simulink model "Control_propulsion_realista"  (R2024b)
settings: Solver=FixedStepAuto  StartTime=0.0  StopTime=tf  FixedStep=50  MaxStep=25  MinStep=1  RelTol=1e-10  AbsTol=1e-10
values from neighbouring files (symbols this model uses):
  v_2 = [-14.5213651902 22.4460020945 10.2931913359]    [datos_trayectoria_mejorada.mat]
undefined symbols (not defined in the file or in its folder): duracion_propul, endDate, F_control, F_quimico, Isp_control, Isp_quimico, m_final, m_i, m_propulsor_quimico, startDate1, ultimo_Tiempo
libraries: simulink x5
settings Model: SimulationMode=rapid-accelerator  Creator=user  LastModifiedBy=benit
settings SolverCC: AutoScaleAbsTol=off  InitialStep=25

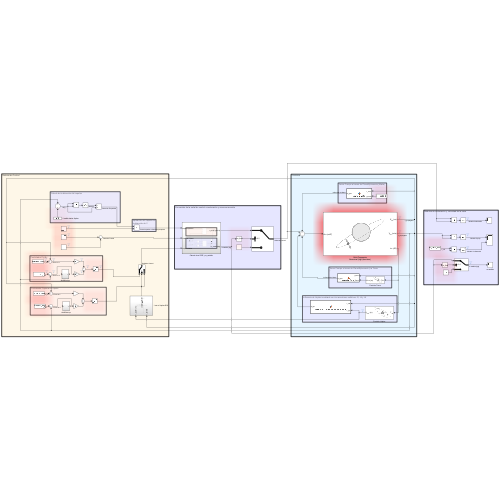
[thumbnail: Simulink's stored preview of the top-level diagram]
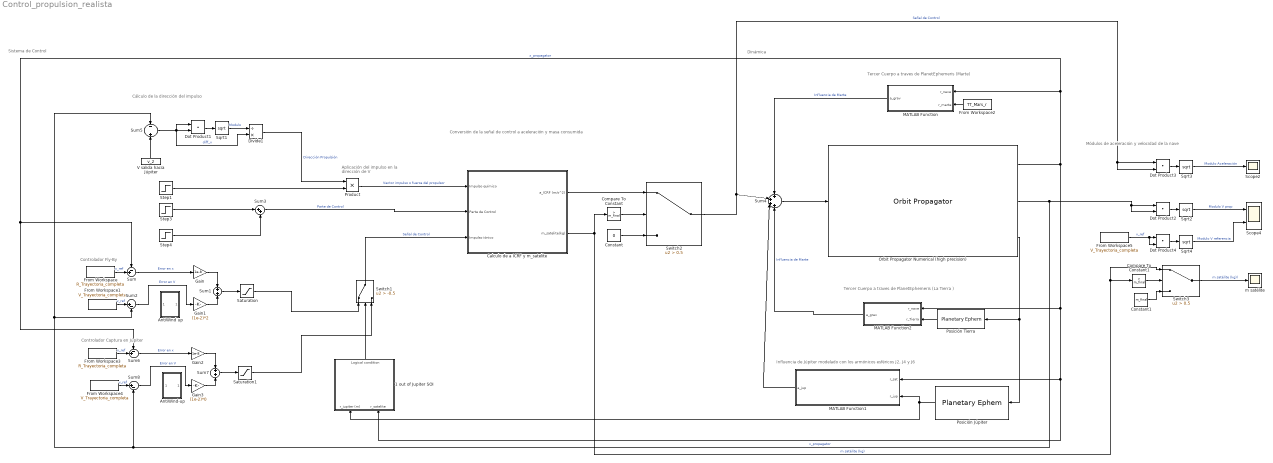
== system Control_propulsion_realista ==
  note: Dinámica
  note: Conversión de la señal de control a aceleración y masa consumida
  note: Sistema de Control
  note: Módulos de aceleración y velocidad de la nave
  note: Controlador Fly-By
  note: Controlador Captura en Júpiter
  note: Influencia de Júpiter modelado con los armónicos esféricos J2, J4 y J6
  note: Cálculo de la dirección del impulso
  note: Tercer Cuerpo a traves de PlanetEphemeris (Marte)
  note: Aplicación del impulso en
      | la dirección de V
  note: Tercer Cuerpo a traves de PlanetEphemeris (La Tierra
      | )
  1 out of Jupiter SOI : Subsystem
  AntiWind up : Subsystem
  AntiWind-up : Subsystem
  Calculo de a ICRF y m_satelite : Subsystem
  Compare To Constant : simulink/Logic and Bit Operations/Compare To Constant  relop=>  const=m_final  OutDataTypeStr=boolean
  Compare To Constant1 : simulink/Logic and Bit Operations/Compare To Constant  relop=>  const=m_final  OutDataTypeStr=boolean
  Constant : Constant  Value=0
  Constant1 : Constant  Value=m_final
  Divide1 : Product  Inputs=/*
  Dot Product{1..4} (4 alike) : DotProduct  OutDataTypeStr=Inherit: Inherit via internal rule
  From Workspace : FromWorkspace  VariableName=R_Trayectoria_completa
  From Workspace1 : FromWorkspace  VariableName=V_Trayectoria_completa
  From Workspace2 : FromWorkspace  VariableName=TT_Mars_r
  From Workspace3 : FromWorkspace  VariableName=R_Trayectoria_completa
  From Workspace4 : FromWorkspace  VariableName=V_Trayectoria_completa
  From Workspace5 : FromWorkspace  VariableName=V_Trayectoria_completa
  Gain : Gain  Gain=1e-8
  Gain1 : Gain  Gain=(1e-2)*2
  Gain2 : Gain  Gain=1e-8
  Gain3 : Gain  Gain=(1e-2)*0
  MATLAB Function : MATLAB Function  TreatAsAtomicUnit=on
  MATLAB Function1 : MATLAB Function  TreatAsAtomicUnit=on
  MATLAB Function2 : MATLAB Function  TreatAsAtomicUnit=on
  Orbit Propagator Numerical (high precision) : OrbitPropagator  propagator=Numerical (high precision)  accelIn=on  startDate=startDate1  semiMajorAxis=sma  eccentricity=ecc  inclination=inc  raan=RAAN  argPeriapsis=aop  trueAnomaly=true_an  inertialPosition=[3649700.0 3308200.0 -4676600.0]  inertialVelocity=[-2750.8 6666.4 2573.4]  fixedPosition=[-4142689.0 -2676864.7 -4669861.6]  fixedVelocity=[1452.7 -6720.7 2568.1]  centralBody=Sun  customR=3396200  customMu=4.305e13  customJ2=1.0826269e-03  customOmega=4.06125949e-3  useEphemerisDateRange=off  ephemerisStartDate=startDate2  ephemerisEndDate=startDate1+tf  includeEarthGravity=off  includeMoonGravity=off  includeJupiterGravity=on
  Posición Júpiter : PlanetaryEphem  units=m,m/s  center=Sun  target=Jupiter  startDate=startDate2  endDate=endDate*1.02  outputVelocity=off
  Posición Tierra : PlanetaryEphem  units=m,m/s  center=Sun  target=Earth  startDate=startDate2  endDate=endDate*1.02  outputVelocity=off
  Product : Product
  Saturation : Saturate  UpperLimit=F_control  LowerLimit=-F_control
  Saturation1 : Saturate  UpperLimit=F_control  LowerLimit=-F_control
  Scope2 : Scope
  Scope4 : Scope  NumInputPorts=2
  Sqrt{1..4} (4 alike) : Sqrt
  Step1 : Step  Time=ultimo_Tiempo+duracion_propul  Before=F_quimico  After=0  SampleTime=0
  Step3 : Step  Time=ultimo_Tiempo  SampleTime=0
  Step4 : Step  Time=ultimo_Tiempo+duracion_propul  After=-1  SampleTime=0
  Sum : Sum  Inputs=-+|
  Sum1 : Sum  Inputs=+|+
  Sum2 : Sum  Inputs=|+-
  Sum3 : Sum  Inputs=|++
  Sum4 : Sum  Inputs=++++
  Sum5 : Sum  Inputs=-+
  Sum6 : Sum  Inputs=-+|
  Sum7 : Sum  Inputs=+|+
  Sum8 : Sum  Inputs=|+-
  Switch1 : Switch  Criteria=u2 > Threshold  Threshold=-0.5  SaturateOnIntegerOverflow=off  InputSameDT=off
  Switch2 : Switch  Criteria=u2 > Threshold  Threshold=0.5  SaturateOnIntegerOverflow=off  InputSameDT=off
  Switch3 : Switch  Criteria=u2 > Threshold  Threshold=0.5  SaturateOnIntegerOverflow=off  InputSameDT=off
  V salida hacia Júpiter : Constant  Value=v_2
  m satélite : Scope
  wires:
  Sum/1 -> Gain/1  "Error en x"
  From Workspace/1 -> Sum/2  "x_ref"
  Orbit Propagator Numerical (high precision)/1 -> Sum6/1, Sum/1, MATLAB Function/1(r_nave), MATLAB Function1/1(r_sat), 1 out of Jupiter SOI/2(r_satelite), MATLAB Function2/1(r_nave)  "x_propagator"
  Gain/1 -> Sum1/1
  From Workspace1/1 -> Sum2/1  "v_ref"
  Gain1/1 -> Sum1/2
  Sum1/1 -> Saturation/1
  Step1/1 -> Product/2
  Step3/1 -> Sum3/1
  Sum4/1 -> Orbit Propagator Numerical (high precision)/1
  Step4/1 -> Sum3/2
  Product/1 -> Calculo de a ICRF y m_satelite/1(Impulso químico)  "Vector impulso o fuerza del propulsor"
  From Workspace2/1 -> MATLAB Function/2(r_marte)
  V salida hacia Júpiter/1 -> Sum5/2
  Sum5/1 -> Dot Product1/1, Divide1/2, Dot Product1/2  "diff_v"
  Sqrt1/1 -> Divide1/1  "Modulo"
  Dot Product1/1 -> Sqrt1/1
  Divide1/1 -> Product/1  "Dirección Propulsión"
  Sum3/1 -> Calculo de a ICRF y m_satelite/2(Parte de Control)  "Parte de Control"
  MATLAB Function/1(a_grav) -> Sum4/1  "Influencia de Marte"
  Orbit Propagator Numerical (high precision)/3 -> Posición Tierra/1, Posición Júpiter/1
  Posición Júpiter/1 -> MATLAB Function1/2(r_jup), 1 out of Jupiter SOI/1(r_jupiter (m))
  From Workspace3/1 -> Sum6/2  "x_ref"
  Sum7/1 -> Saturation1/1
  From Workspace4/1 -> Sum8/1  "v_ref"
  Gain2/1 -> Sum7/1
  Gain3/1 -> Sum7/2
  Sum6/1 -> Gain2/1  "Error en x"
  Orbit Propagator Numerical (high precision)/2 -> Dot Product2/2, Dot Product2/1, Sum2/2, Sum5/1, Sum8/2  "v_propagator"
  Saturation/1 -> Switch1/1
  Saturation1/1 -> Switch1/3
  Switch1/1 -> Calculo de a ICRF y m_satelite/3(Impulso iónico)  "Señal de Control"
  Calculo de a ICRF y m_satelite/2(m_satelite(kg)) -> Switch3/1, Compare To Constant1/1, Compare To Constant/1  "m satélite (kg)"
  Dot Product2/1 -> Sqrt2/1
  Sqrt2/1 -> Scope4/1  "Modulo V prop"
  Sqrt3/1 -> Scope2/1  "Modulo Aceleración"
  Dot Product3/1 -> Sqrt3/1
  Sqrt4/1 -> Scope4/2  "Modulo V referencia"
  Dot Product4/1 -> Sqrt4/1
  From Workspace5/1 -> Dot Product4/2, Dot Product4/1  "v_ref"
  MATLAB Function1/1(a_jup) -> Sum4/3
  Switch2/1 -> Dot Product3/2, Dot Product3/1, Sum4/2  "Señal de Control"
  Calculo de a ICRF y m_satelite/1(a_ICRF (m/s^2)) -> Switch2/1
  Constant/1 -> Switch2/3
  Compare To Constant/1 -> Switch2/2
  Compare To Constant1/1 -> Switch3/2
  Constant1/1 -> Switch3/3
  Switch3/1 -> m satélite/1  "m satélite (kg)l"
  1 out of Jupiter SOI/1("Logical condition ") -> Switch1/2
  Posición Tierra/1 -> MATLAB Function2/2(r_Tierra)
  Sum2/1 -> Gain1/1  "Error en V"
  Sum8/1 -> Gain3/1  "Error en V"
  MATLAB Function2/1(a_grav) -> Sum4/4  "Influencia de Marte"

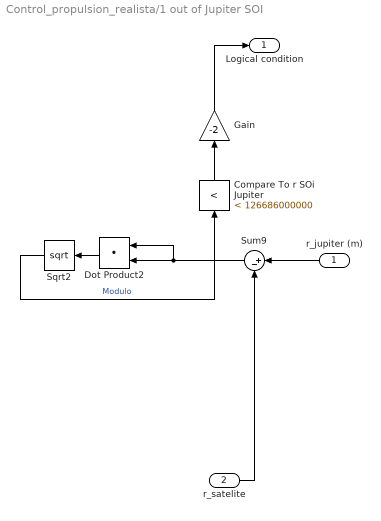
== system Control_propulsion_realista/1 out of Jupiter SOI ==
  r_jupiter (m) : Inport
  r_satelite : Inport  Port=2
  Compare To r SOi Jupiter : simulink/Logic and Bit Operations/Compare To Constant  relop=<  const=126686000000  OutDataTypeStr=boolean
  Dot Product2 : DotProduct  OutDataTypeStr=Inherit: Inherit via internal rule
  Gain : Gain  Gain=-2
  Sqrt2 : Sqrt
  Sum9 : Sum  Inputs=|+-
  "Logical condition " : Outport
  wires:
  Dot Product2/1 -> Sqrt2/1
  r_satelite/1 -> Sum9/2
  Compare To r SOi Jupiter/1 -> Gain/1
  Sqrt2/1 -> Compare To r SOi Jupiter/1  "Modulo"
  r_jupiter (m)/1 -> Sum9/1
  Sum9/1 -> Dot Product2/2, Dot Product2/1
  Gain/1 -> "Logical condition "/1

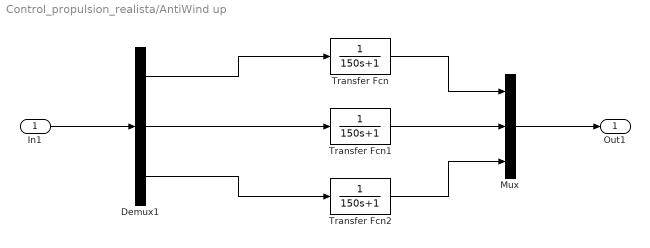
== system Control_propulsion_realista/AntiWind up ==
  In1 : Inport
  Demux1 : Demux  Outputs=3
  Mux : Mux  Inputs=3
  Transfer Fcn : TransferFcn  Denominator=[150 1]
  Transfer Fcn1 : TransferFcn  Denominator=[150 1]
  Transfer Fcn2 : TransferFcn  Denominator=[150 1]
  Out1 : Outport
  wires:
  Demux1/1 -> Transfer Fcn/1
  Demux1/2 -> Transfer Fcn1/1
  Demux1/3 -> Transfer Fcn2/1
  Transfer Fcn/1 -> Mux/1
  Transfer Fcn1/1 -> Mux/2
  Transfer Fcn2/1 -> Mux/3
  Mux/1 -> Out1/1
  In1/1 -> Demux1/1

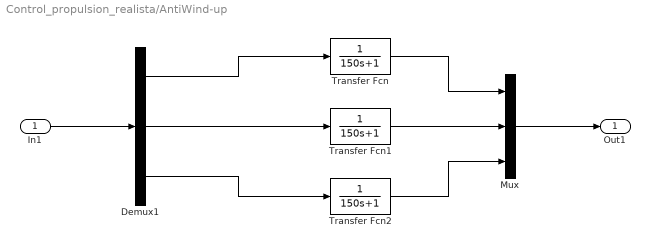
== system Control_propulsion_realista/AntiWind-up ==
  In1 : Inport
  Demux1 : Demux  Outputs=3
  Mux : Mux  Inputs=3
  Transfer Fcn : TransferFcn  Denominator=[150 1]
  Transfer Fcn1 : TransferFcn  Denominator=[150 1]
  Transfer Fcn2 : TransferFcn  Denominator=[150 1]
  Out1 : Outport
  wires:
  Demux1/1 -> Transfer Fcn/1
  Demux1/2 -> Transfer Fcn1/1
  Demux1/3 -> Transfer Fcn2/1
  Transfer Fcn/1 -> Mux/1
  Transfer Fcn1/1 -> Mux/2
  Transfer Fcn2/1 -> Mux/3
  Mux/1 -> Out1/1
  In1/1 -> Demux1/1

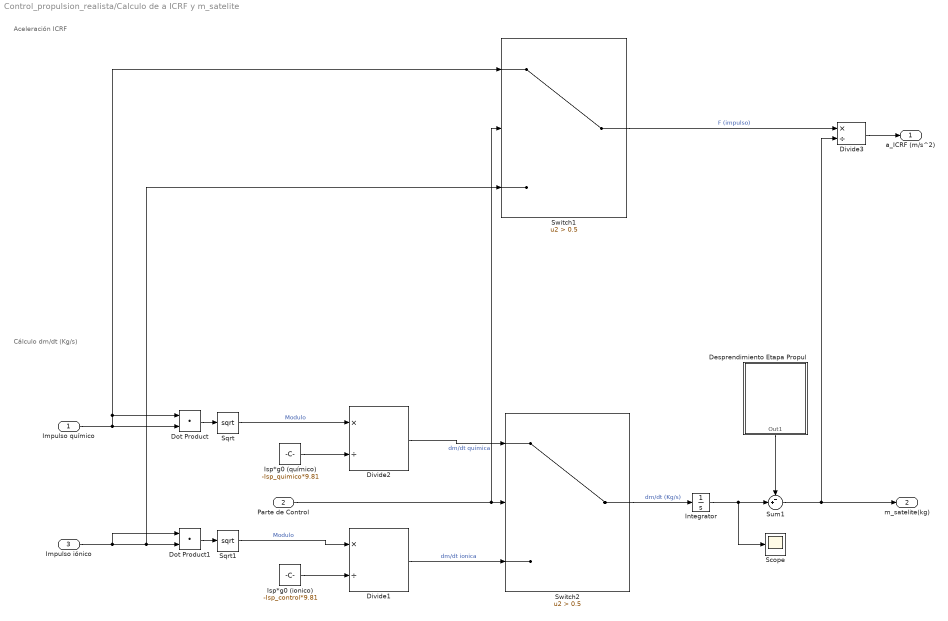
== system Control_propulsion_realista/Calculo de a ICRF y m_satelite ==
  note: Aceleración ICRF
  note: Cálculo dm/dt (Kg/s)
  Impulso químico : Inport
  Parte de Control : Inport  Port=2
  Impulso iónico : Inport  Port=3
  Desprendimiento Etapa Propul : Subsystem
  Divide1 : Product  Inputs=*/
  Divide2 : Product  Inputs=*/
  Divide3 : Product  Inputs=*/
  Dot Product : DotProduct  OutDataTypeStr=Inherit: Inherit via internal rule
  Dot Product1 : DotProduct  OutDataTypeStr=Inherit: Inherit via internal rule
  Integrator : Integrator  InitialCondition=m_i
  Isp*g0 (ionico) : Constant  Value=-Isp_control*9.81
  Isp*g0 (químico) : Constant  Value=-Isp_quimico*9.81
  Scope : Scope
  Sqrt : Sqrt
  Sqrt1 : Sqrt
  Sum1 : Sum  Inputs=-+|
  Switch1 : Switch  Criteria=u2 > Threshold  Threshold=0.5  SaturateOnIntegerOverflow=off  InputSameDT=off
  Switch2 : Switch  Criteria=u2 > Threshold  Threshold=0.5  SaturateOnIntegerOverflow=off  InputSameDT=off
  a_ICRF (m/s^2) : Outport
  m_satelite(kg) : Outport  Port=2
  wires:
  Parte de Control/1 -> Switch1/2, Switch2/2
  Divide2/1 -> Switch2/1  "dm/dt química"
  Isp*g0 (químico)/1 -> Divide2/2
  Isp*g0 (ionico)/1 -> Divide1/2
  Divide1/1 -> Switch2/3  "dm/dt ionica"
  Switch2/1 -> Integrator/1  "dm/dt (Kg/s)"
  Dot Product/1 -> Sqrt/1
  Impulso químico/1 -> Switch1/1, Dot Product/1, Dot Product/2
  Sqrt/1 -> Divide2/1  "Modulo"
  Dot Product1/1 -> Sqrt1/1
  Sqrt1/1 -> Divide1/1  "Modulo"
  Impulso iónico/1 -> Switch1/3, Dot Product1/2, Dot Product1/1
  Switch1/1 -> Divide3/1  "F (impulso)"
  Divide3/1 -> a_ICRF (m/s^2)/1
  Integrator/1 -> Scope/1, Sum1/2
  Desprendimiento Etapa Propul/1(Out1) -> Sum1/1
  Sum1/1 -> Divide3/2, m_satelite(kg)/1

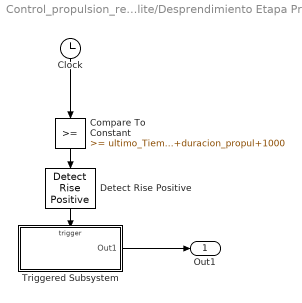
== system Control_propulsion_realista/Calculo de a ICRF y m_satelite/Desprendimiento Etapa Propul ==
  Clock : Clock
  Compare To Constant : simulink/Logic and Bit Operations/Compare To Constant  relop=>=  const=ultimo_Tiempo+duracion_propul+1000  OutDataTypeStr=boolean
  Detect Rise Positive : simulink/Logic and Bit Operations/Detect Rise Positive  vinit=0  OutDataTypeStr=boolean
  Triggered Subsystem : Subsystem  TreatAsAtomicUnit=on
  Out1 : Outport
  wires:
  Clock/1 -> Compare To Constant/1
  Detect Rise Positive/1 -> Triggered Subsystem/Trigger
  Compare To Constant/1 -> Detect Rise Positive/1
  Triggered Subsystem/1(Out1) -> Out1/1

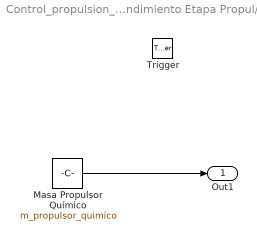
== system Control_propulsion_realista/Calculo de a ICRF y m_satelite/Desprendimiento Etapa Propul/Triggered Subsystem ==
  Trigger : TriggerPort  VariantControl=(inherit)
  Masa Propulsor Químico : Constant  Value=m_propulsor_quimico
  Out1 : Outport
  wires:
  Masa Propulsor Químico/1 -> Out1/1

== matlab function Control_propulsion_realista/MATLAB Function ==
  data: r_nave input; a_grav output; r_marte input
function a_grav = gravedadMarte(r_nave, r_marte)
%#codegen

% Constante gravitacional de Marte
mu_marte = 4.282837e13; % [m^3/s^2]

% Vector relativo
r_rel = r_nave - r_marte;

% Magnitud de la distancia
dist = norm(r_rel);

% Aceleración gravitatoria
a_grav = (-mu_marte / dist^3) * r_rel;

end

== matlab function Control_propulsion_realista/MATLAB Function2 ==
  data: r_nave input; a_grav output; r_Tierra input
function a_grav = gravedadTierra(r_nave, r_Tierra)
%#codegen

% Constante gravitacional de Marte
mu_marte = 3.986e14; % [m^3/s^2]

% Vector relativo
r_rel = r_nave - r_Tierra;

% Magnitud de la distancia
dist = norm(r_rel);

% Aceleración gravitatoria
a_grav = (-mu_marte / dist^3) * r_rel;

end

== matlab function Control_propulsion_realista/MATLAB Function1 ==
  data: r_sat input; a_jup output; r_jup input
function a_jup = aceleracion_jupiter_armonicos_simulink(r_sat, r_jup)
    % Entradas y salidas en metros / segundos
    % r_sat, r_jup: [3x1] vectores de posición en metros

    % Constantes de Júpiter (SI)
    mu_jup = 1.26686534e17;    % m^3/s^2
    R_jup = 71492e3;           % m

    % Coeficientes zonales (J2, J4, J6) adimensionales
    J = [0.0146965735, -0.00058722, 0.0000342];

    % Posición relativa
    r_rel = r_sat - r_jup;
    x = r_rel(1); y = r_rel(2); z = r_rel(3);
    r = sqrt(x^2 + y^2 + z^2);
    u = z / r;

    % Aceleración central
    a_central = -mu_jup / r^3 * r_rel;

    % Inicializar aceleración zonal
    a_J = zeros(3,1);

    % Evaluar cada término armónico
    for n = [2, 4, 6]
        idx = n / 2;

         % Inicialización obligatoria para evitar errores de compilación
         Pn = 0;
         dP = 0;
        % Evaluar Pn(u) y Pn'(u)
        switch n
            case 2
                Pn = 0.5 * (3*u^2 - 1);
                dP = 3*u;
            case 4
                Pn = (1/8) * (35*u^4 - 30*u^2 + 3);
                dP = 0.5 * (140*u^3 - 60*u);
            case 6
                Pn = (1/16) * (231*u^6 - 315*u^4 + 105*u^2 - 5);
                dP = (1/16) * (1386*u^5 - 1260*u^3 + 210*u);
        end

        % Derivadas del potencial
        r_ratio = (R_jup / r)^n;
        factor = mu_jup * r_ratio * J(idx) / r^2;
        dU_dr = factor * (n + 1) * Pn;
        dU_du = factor * dP;

        % Aceleración en coordenadas cartesianas
        a_r = -dU_dr;
        a_u = dU_du;

        % Transformación de derivadas a aceleración cartesiana
        a_J = a_J + (a_r * r_rel / r) + ...
              a_u * ( (z / r^2) * r_rel - [0; 0; 1] );
    end

    % Aceleración total (en m/s^2)
    a_jup = a_central + a_J;
end
